simulink model "SkywalkerX8_Lateral_Control_Digital_Verification"  (R2018a)
settings: Solver=FixedStepAuto  StartTime=0.0  StopTime=30  FixedStep=0.001  RelTol=1e-3
undefined symbols (not defined in the file): DiscIntNeverNeededParam, sigbuilder_block, SkywalkerX8
libraries: simulink_extras x11, simulink x1
settings Model: SnapshotBufferSize=1000  SnapshotInterval=1  Creator=David  LastModifiedBy=David

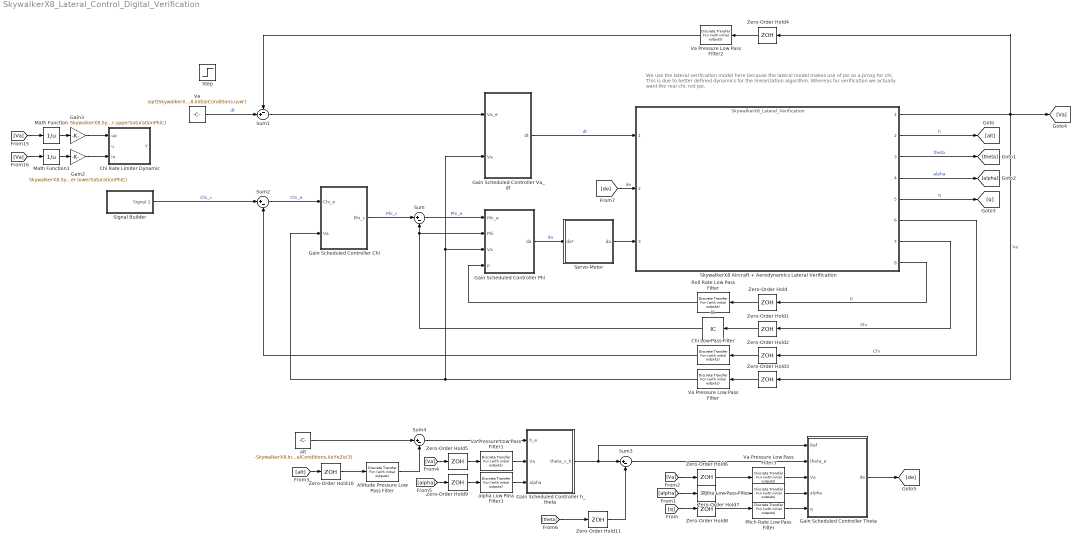
== system SkywalkerX8_Lateral_Control_Digital_Verification ==
  note: We use the lateral verification model here because the lateral model makes use of psi as a proxy for chi.
      | This is due to better defined dynamics for the linearization algorithm. Whereas for verification we actually
      | want the real chi, not psi.
  Altitude Pressure Low Pass Filter : simulink_extras/Additional Discrete/Discrete Transfer Fcn (with initial outputs)  N=cell2mat(SkywalkerX8.Sensors.Filters.AltitudePressure.FilterTFDigital.Numerator)  D=cell2mat(SkywalkerX8.Sensors.Filters.AltitudePressure.FilterTFDigital.Denominator)  U0=-SkywalkerX8.InitialConditions.XeYeZe(3)  Y0=-SkywalkerX8.InitialConditions.XeYeZe(3)  TS=SkywalkerX8.Sensors.Filters.AltitudePressure.FilterSampleTime
      settings: SourceProductName=Simulink  SourceProductBaseCode=SL
  Chi Low Pass Filter : simulink_extras/Additional Discrete/Discrete Transfer Fcn (with initial outputs)  N=cell2mat(SkywalkerX8.Sensors.EKF.GPSSmoothing.Filters.ChiFilter.TFDigital.Numerator)  D=cell2mat(SkywalkerX8.Sensors.EKF.GPSSmoothing.Filters.ChiFilter.TFDigital.Denominator)  U0=SkywalkerX8.Sensors.EKF.GPSSmoothing.Filters.ChiFilter.InitialCondition  Y0=SkywalkerX8.Sensors.EKF.GPSSmoothing.Filters.ChiFilter.InitialCondition  TS=SkywalkerX8.Sensors.EKF.GPSSmoothing.Filters.ChiFilter.SampleTime
      settings: SourceProductName=Simulink  SourceProductBaseCode=SL
  Chi Rate Limiter Dynamic : Subsystem  mask{initOutput=SkywalkerX8.InitialConditions.PhiThetaPsi(3)}
      mask prompts: initOutput "Initial output of dynamic rate limiter"
      mask DialogControl DescGroupVar Prompt: Rate Limiter Dynamic
      mask DialogControl DescTextVar Prompt: Limit rising and falling rates of the signals at the second input by using the first input (upper limit) and the third input (lower limit).
      mask Display:
      | image('rateLimit.png')
      | 
      | port_label('input', 1, 'up')
      | port_label('input', 2, 'u')
      | port_label('input', 3, 'lo')
      | 
      | port_label('output', 1, 'Y')
  Gain Scheduled Controller Chi : Subsystem
  Gain Scheduled Controller Phi : Subsystem
  Gain Scheduled Controller Theta : Subsystem
  Gain Scheduled Controller Va_dt : Subsystem
  Gain Scheduled Controller h_theta : Subsystem
  Gain2 : Gain  Gain=SkywalkerX8.System.Gravity*tan(0.75*SkywalkerX8.Control.Lateral.ChiController.lowerSaturationPhiC)
  Gain3 : Gain  Gain=SkywalkerX8.System.Gravity*tan(0.75*SkywalkerX8.Control.Lateral.ChiController.upperSaturationPhiC)
  IC : InitialCondition  Value=SkywalkerX8.InitialConditions.PhiThetaPsi(1)
  Math Function : Math  Operator=reciprocal  SaturateOnIntegerOverflow=on
  Math Function1 : Math  Operator=reciprocal  SaturateOnIntegerOverflow=on
  Pitch Rate Low Pass Filter : simulink_extras/Additional Discrete/Discrete Transfer Fcn (with initial outputs)  N=cell2mat(SkywalkerX8.Sensors.Filters.AngularRates.Pitch.FilterTFDigital.Numerator)  D=cell2mat(SkywalkerX8.Sensors.Filters.AngularRates.Pitch.FilterTFDigital.Denominator)  U0=SkywalkerX8.Sensors.Filters.AngularRates.Pitch.InitialCondition  Y0=SkywalkerX8.Sensors.Filters.AngularRates.Pitch.InitialCondition  TS=SkywalkerX8.Sensors.Filters.AngularRates.Pitch.FilterSampleTime
      settings: SourceProductName=Simulink  SourceProductBaseCode=SL
  Roll Rate Low Pass Filter : simulink_extras/Additional Discrete/Discrete Transfer Fcn (with initial outputs)  N=cell2mat(SkywalkerX8.Sensors.Filters.AngularRates.Roll.FilterTFDigital.Numerator)  D=cell2mat(SkywalkerX8.Sensors.Filters.AngularRates.Roll.FilterTFDigital.Denominator)  U0=SkywalkerX8.Sensors.Filters.AngularRates.Roll.InitialCondition  Y0=SkywalkerX8.Sensors.Filters.AngularRates.Roll.InitialCondition  TS=SkywalkerX8.Sensors.Filters.AngularRates.Roll.FilterSampleTime
      settings: SourceProductName=Simulink  SourceProductBaseCode=SL
  Servo-Motor : Subsystem
      mask Display: image('servo.jpg', 'center')
  Signal Builder : Subsystem  Tag=STV Subsys  LoadFcn=sigbuilder_block('load');  StartFcn=sigbuilder_block('start');  StopFcn=sigbuilder_block('stop');  ClipboardFcn=sigbuilder_block('clipboard');  mask(Sigbuilder block){tuvar=[0:10]}
      mask help: Simulink:masks:SigbuilderBlock_MD
      mask init:
      | if ~strcmp(get_param(bdroot(gcbh),'SimulationStatus'),'stopped') tuvar = sigbuilder_block('maskInit'); end
      settings: CopyFcn=sigbuilder_block('copy');  DeleteFcn=sigbuilder_block('delete');  ModelCloseFcn=sigbuilder_block('modelClose');  PreSaveFcn=sigbuilder_block('preSave');  PauseFcn=sigbuilder_block('pause');  ContinueFcn=sigbuilder_block('continue');  NameChangeFcn=sigbuilder_block('namechange');  OpenFcn=sigbuilder_block('open',[437.6 199.2 550.4 400 ]);  CloseFcn=sigbuilder_block('close');
      mask Display: plot(0, 0, 100, 100,[2, 2, 32, 32, 2], [68, 8, 8, 68, 68],[32, 2], [38, 38], [32, 19, 2],[53, 60, 44], [32, 17, 17, 2],[16, 16, 31, 31]);txt = getActiveGroup(gcbh);text(2, 100, txt,'verticalAlignment', 'top');
  SkywalkerX8 Aircraft + Aerodynamics Lateral Verification : ModelReference  ModelNameDialog=SkywalkerX8_Lateral_Verification.slx  ModelReferenceVersion=1.41
      mask Display:
      | image('x8SkySunset.png', 'center')
      | 
      | port_label('input', 1, '\delta_t (Unitless)', 'texmode', 'on')
      | port_label('input', 2, '\delta_e (rad)', 'texmode', 'on')
      | port_label('input', 3, '\delta_a (rad)', 'texmode', 'on')
      | 
      | port_label('output', 1, 'V_a (m/s)', 'texmode', 'on')
      | port_label('output', 2, 'Altitude (m)', 'texmode', 'on')
      | port_label('output', 3, '\theta (rad)', 'texmode', 'on')
      | port_label('output', 4, 'alpha (rad)', 'texmode', 'on')
      | port_label('output', 5, 'q (rad/s)', 'texmode', 'on')
      | port_label('output', 6, '\chi (rad)', 'texmode', 'on')
      | port_label('output', 7, '\Phi (rad)', 'texmode', 'on')
      | port_label('output', 8, 'p (rad/s)', 'texmode', 'on')
  Step : Step  After=deg2rad(90)  SampleTime=0
  Sum{,2..4} (4 alike) : Sum  Inputs=|+-
  Sum1 : Sum  Inputs=-+|
  Va : Constant  Value=sqrt(SkywalkerX8.InitialConditions.uvw*SkywalkerX8.InitialConditions.uvw')
  Va Pressure Low Pass Filter{,1..3} (4 alike) : simulink_extras/Additional Discrete/Discrete Transfer Fcn (with initial outputs)  N=cell2mat(SkywalkerX8.Sensors.Filters.AirspeedPressure.FilterTFDigital.Numerator)  D=cell2mat(SkywalkerX8.Sensors.Filters.AirspeedPressure.FilterTFDigital.Denominator)  U0=sqrt(SkywalkerX8.InitialConditions.uvw*SkywalkerX8.InitialConditions.uvw')  Y0=SkywalkerX8.Sensors.Filters.AirspeedPressure.InitialCondition  TS=SkywalkerX8.Sensors.Filters.AirspeedPressure.FilterSampleTime
      settings: SourceProductName=Simulink  SourceProductBaseCode=SL
  Zero-Order Hold : ZeroOrderHold  SampleTime=SkywalkerX8.Sensors.IMU.Gyroscope.SampleTime
  Zero-Order Hold1 : ZeroOrderHold  SampleTime=SkywalkerX8.Sensors.EKF.Attitude.StateTransitionSampleTime
  Zero-Order Hold10 : ZeroOrderHold  SampleTime=SkywalkerX8.Sensors.AltitudePressure.SampleTime
  Zero-Order Hold11 : ZeroOrderHold  SampleTime=SkywalkerX8.Sensors.EKF.GPSSmoothing.StateTransitionSampleTime
  Zero-Order Hold2 : ZeroOrderHold  SampleTime=SkywalkerX8.Sensors.EKF.GPSSmoothing.MeasurementSampleTime
  Zero-Order Hold{3..6} (4 alike) : ZeroOrderHold  SampleTime=SkywalkerX8.Sensors.AirspeedPressure.SampleTime
  Zero-Order Hold7 : ZeroOrderHold  SampleTime=SkywalkerX8.Sensors.AoA.SampleTime
  Zero-Order Hold8 : ZeroOrderHold  SampleTime=SkywalkerX8.Sensors.IMU.Gyroscope.SampleTime
  Zero-Order Hold9 : ZeroOrderHold  SampleTime=SkywalkerX8.Sensors.AoA.SampleTime
  alpha Low Pass Filter : simulink_extras/Additional Discrete/Discrete Transfer Fcn (with initial outputs)  N=cell2mat(SkywalkerX8.Sensors.Filters.AoA.FilterTFDigital.Numerator)  D=cell2mat(SkywalkerX8.Sensors.Filters.AoA.FilterTFDigital.Denominator)  U0=SkywalkerX8.Sensors.Filters.AoA.InitialCondition  Y0=SkywalkerX8.Sensors.Filters.AoA.InitialCondition  TS=SkywalkerX8.Sensors.Filters.AoA.FilterSampleTime
      settings: SourceProductName=Simulink  SourceProductBaseCode=SL
  alpha Low Pass Filter1 : simulink_extras/Additional Discrete/Discrete Transfer Fcn (with initial outputs)  N=cell2mat(SkywalkerX8.Sensors.Filters.AoA.FilterTFDigital.Numerator)  D=cell2mat(SkywalkerX8.Sensors.Filters.AoA.FilterTFDigital.Denominator)  U0=SkywalkerX8.Sensors.Filters.AoA.InitialCondition  Y0=SkywalkerX8.Sensors.Filters.AoA.InitialCondition  TS=SkywalkerX8.Sensors.Filters.AoA.FilterSampleTime
      settings: SourceProductName=Simulink  SourceProductBaseCode=SL
  alt : Constant  Value=-SkywalkerX8.InitialConditions.XeYeZe(3)
  wires:
  SkywalkerX8 Aircraft + Aerodynamics Lateral Verification/7 -> Zero-Order Hold1/1  "Phi"
  SkywalkerX8 Aircraft + Aerodynamics Lateral Verification/1 -> [Va], Zero-Order Hold3/1, Zero-Order Hold4/1  "Va"
  Gain Scheduled Controller Chi/1(Phi_c) -> Sum/1  "Phi_c"
  Sum/1 -> Gain Scheduled Controller Phi/1(Phi_e)  "Phi_e"
  Sum2/1 -> Gain Scheduled Controller Chi/1(Chi_e)  "Chi_e"
  SkywalkerX8 Aircraft + Aerodynamics Lateral Verification/8 -> Zero-Order Hold/1  "p"
  Gain Scheduled Controller Phi/1(da) -> Servo-Motor/1(da*)  "da"
  [de] -> SkywalkerX8 Aircraft + Aerodynamics Lateral Verification/2  "de"
  Gain Scheduled Controller Va_dt/1(dt) -> SkywalkerX8 Aircraft + Aerodynamics Lateral Verification/1  "dt"
  SkywalkerX8 Aircraft + Aerodynamics Lateral Verification/6 -> Zero-Order Hold2/1  "Chi"
  Va/1 -> Sum1/2  "dt"
  Sum1/1 -> Gain Scheduled Controller Va_dt/1(Va_e)
  Gain Scheduled Controller h_theta/1(theta_c_h) -> Gain Scheduled Controller Theta/1(Ref), Sum3/1
  Sum3/1 -> Gain Scheduled Controller Theta/2(theta_e)
  SkywalkerX8 Aircraft + Aerodynamics Lateral Verification/2 -> [alt]  "h"
  SkywalkerX8 Aircraft + Aerodynamics Lateral Verification/3 -> [theta]  "theta"
  SkywalkerX8 Aircraft + Aerodynamics Lateral Verification/4 -> [alpha]  "alpha"
  SkywalkerX8 Aircraft + Aerodynamics Lateral Verification/5 -> [q]  "q"
  [q] -> Zero-Order Hold8/1
  [alpha] -> Zero-Order Hold7/1
  [Va] -> Zero-Order Hold6/1
  Sum4/1 -> Gain Scheduled Controller h_theta/1(h_e)
  [alt] -> Zero-Order Hold10/1
  alt/1 -> Sum4/1
  [Va] -> Zero-Order Hold5/1
  [alpha] -> Zero-Order Hold9/1
  [theta] -> Zero-Order Hold11/1
  Gain Scheduled Controller Theta/1(de) -> [de]
  Servo-Motor/1(da) -> SkywalkerX8 Aircraft + Aerodynamics Lateral Verification/3
  Zero-Order Hold/1 -> Roll Rate Low Pass Filter/1
  Zero-Order Hold1/1 -> IC/1
  Zero-Order Hold2/1 -> Chi Low Pass Filter/1
  Zero-Order Hold3/1 -> Va Pressure Low Pass Filter/1
  Zero-Order Hold4/1 -> Va Pressure Low Pass Filter2/1
  Zero-Order Hold5/1 -> Va Pressure Low Pass Filter1/1
  Zero-Order Hold6/1 -> Va Pressure Low Pass Filter3/1
  Zero-Order Hold7/1 -> alpha Low Pass Filter/1
  Zero-Order Hold8/1 -> Pitch Rate Low Pass Filter/1
  Zero-Order Hold9/1 -> alpha Low Pass Filter1/1
  Zero-Order Hold10/1 -> Altitude Pressure Low Pass Filter/1
  Zero-Order Hold11/1 -> Sum3/2
  Roll Rate Low Pass Filter/1 -> Gain Scheduled Controller Phi/4(p)
  Chi Low Pass Filter/1 -> Sum2/2
  Va Pressure Low Pass Filter/1 -> Gain Scheduled Controller Chi/2(Va), Gain Scheduled Controller Va_dt/2(Va), Gain Scheduled Controller Phi/3(Va)
  Pitch Rate Low Pass Filter/1 -> Gain Scheduled Controller Theta/5(q)
  alpha Low Pass Filter/1 -> Gain Scheduled Controller Theta/4(alpha)
  Altitude Pressure Low Pass Filter/1 -> Sum4/2
  Va Pressure Low Pass Filter1/1 -> Gain Scheduled Controller h_theta/2(Va)
  alpha Low Pass Filter1/1 -> Gain Scheduled Controller h_theta/3(alpha)
  Va Pressure Low Pass Filter2/1 -> Sum1/1
  Va Pressure Low Pass Filter3/1 -> Gain Scheduled Controller Theta/3(Va)
  IC/1 -> Gain Scheduled Controller Phi/2(Phi), Sum/2
  [Va] -> Math Function/1
  Math Function1/1 -> Gain2/1
  Gain2/1 -> Chi Rate Limiter Dynamic/3(lo)
  Math Function/1 -> Gain3/1
  Gain3/1 -> Chi Rate Limiter Dynamic/1(up)
  [Va] -> Math Function1/1
  Signal Builder/1(Signal 1) -> Sum2/1  "Chi_c"

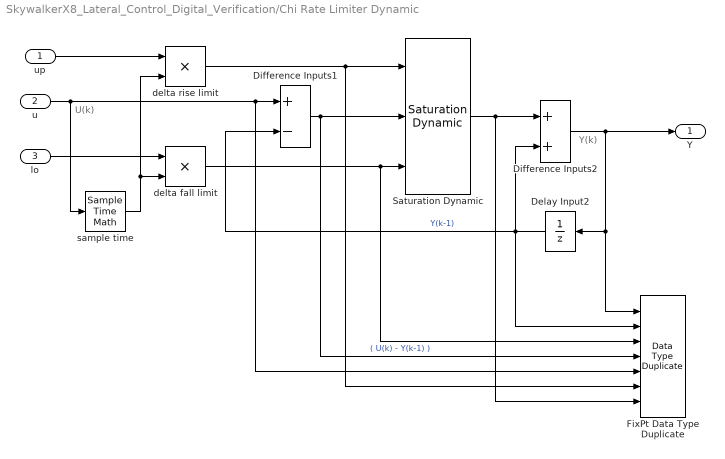
== system SkywalkerX8_Lateral_Control_Digital_Verification/Chi Rate Limiter Dynamic ==
  note: U(k)
  note: Y(k)
  up : Inport
  u : Inport  Port=2
  lo : Inport  Port=3
  Delay Input2 : UnitDelay  Description=Store in Global RAM  DisableCoverage=on  InitialCondition=initOutput  SampleTime=-1
  Difference Inputs1 : Sum  Description=Add in CPU  DisableCoverage=on  Inputs=+-  OutDataTypeStr=Inherit: Inherit via back propagation
  Difference Inputs2 : Sum  Description=Add in CPU  OutDataTypeStr=Inherit: Inherit via back propagation
  FixPt Data Type Duplicate : DataTypeDuplicate  DisableCoverage=on  NumInputPorts=7
  Saturation Dynamic : simulink/Discontinuities/Saturation Dynamic  OutMin=[]  OutMax=[]  OutDataTypeStr=Inherit: Same as second input  OutDataType=fixdt(1, 16)  OutScaling=2^-10  DoSatur=off
  delta fall limit : Product  DisableCoverage=on  Inputs=**  OutDataTypeStr=Inherit: Inherit via back propagation  SaturateOnIntegerOverflow=on
  delta rise limit : Product  DisableCoverage=on  Inputs=**  OutDataTypeStr=Inherit: Inherit via back propagation  SaturateOnIntegerOverflow=on
  sample time : SampleTimeMath  DisableCoverage=on  TsampMathOp=Ts Only  weightValue=1
  Y : Outport  InitialOutput=0
  wires:
  Delay Input2/1 -> Difference Inputs1/2, FixPt Data Type Duplicate/2, Difference Inputs2/2  "Y(k-1)"
  Difference Inputs1/1 -> FixPt Data Type Duplicate/4, Saturation Dynamic/2  "( U(k) - Y(k-1) )"
  Difference Inputs2/1 -> Y/1, Delay Input2/1, FixPt Data Type Duplicate/1
  u/1 -> Difference Inputs1/1, FixPt Data Type Duplicate/5, sample time/1
  delta fall limit/1 -> FixPt Data Type Duplicate/3, Saturation Dynamic/3
  sample time/1 -> delta fall limit/2, delta rise limit/2
  Saturation Dynamic/1 -> Difference Inputs2/1, FixPt Data Type Duplicate/7
  delta rise limit/1 -> FixPt Data Type Duplicate/6, Saturation Dynamic/1
  lo/1 -> delta fall limit/1
  up/1 -> delta rise limit/1

== system SkywalkerX8_Lateral_Control_Digital_Verification/Gain Scheduled Controller Chi ==
  Chi_e : Inport
  Va : Inport  Port=2
  PIDF Controller Chi Ki 2D Lookup Table : Lookup_n-D  NumberOfTableDimensions=1  BreakpointsForDimension1=SkywalkerX8.Control.Lateral.SchedulingVariables.VaArray  BreakpointsForDimension2=SkywalkerX8.Control.Longitudinal.SchedulingVariables.alphaArray  Table=SkywalkerX8.Control.Lateral.ChiController.Digital.KiChi  InternalRulePriority=Speed  RndMeth=Simplest  InputSameDT=on
  PIDF Controller Chi Kp 2D Lookup Table : Lookup_n-D  NumberOfTableDimensions=1  BreakpointsForDimension1=SkywalkerX8.Control.Lateral.SchedulingVariables.VaArray  BreakpointsForDimension2=SkywalkerX8.Control.Longitudinal.SchedulingVariables.alphaArray  Table=SkywalkerX8.Control.Lateral.ChiController.Digital.KpChi  InternalRulePriority=Speed  RndMeth=Simplest  InputSameDT=on
  PIDF Controller Va_theta : Subsystem
  Saturation : Saturate  UpperLimit=SkywalkerX8.Control.Lateral.ChiController.upperSaturationPhiC  LowerLimit=SkywalkerX8.Control.Lateral.ChiController.lowerSaturationPhiC
  Phi_c : Outport
  wires:
  PIDF Controller Chi Kp 2D Lookup Table/1 -> PIDF Controller Va_theta/2(P)
  Chi_e/1 -> PIDF Controller Va_theta/1(u)
  Va/1 -> PIDF Controller Chi Kp 2D Lookup Table/1, PIDF Controller Chi Ki 2D Lookup Table/1
  PIDF Controller Chi Ki 2D Lookup Table/1 -> PIDF Controller Va_theta/3(I)
  Saturation/1 -> PIDF Controller Va_theta/4(Post-Saturation), Phi_c/1
  PIDF Controller Va_theta/1(y) -> PIDF Controller Va_theta/5(Pre-Saturation), Saturation/1

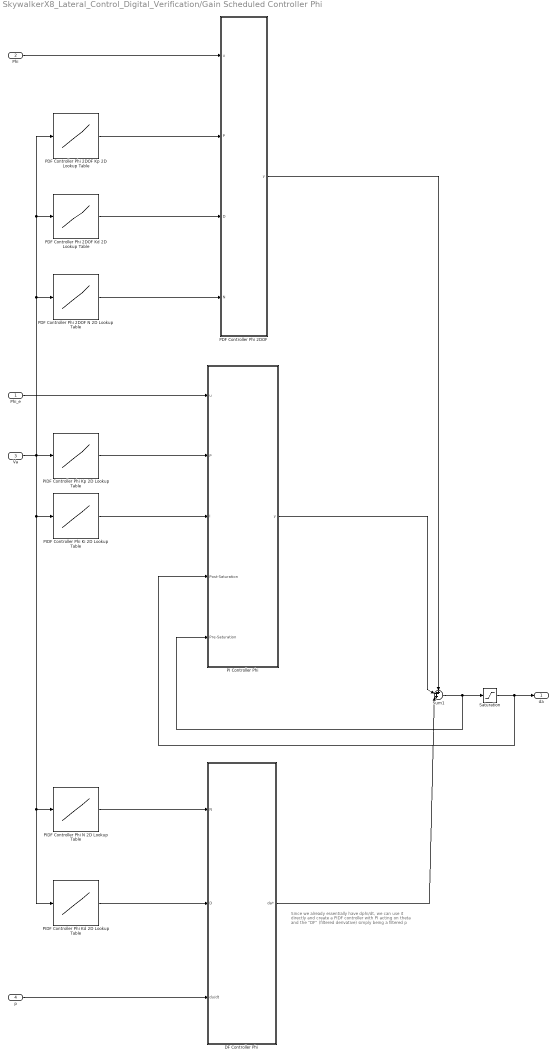
== system SkywalkerX8_Lateral_Control_Digital_Verification/Gain Scheduled Controller Phi ==
  note: Since we already essentially have dphi/dt,
      | we can use it directly and create a PIDF controller
      | with PI acting on theta and the "DF" (filtered derivative)
      | simply being a filtered p
  Phi_e : Inport
  Phi : Inport  Port=2
  Va : Inport  Port=3
  p : Inport  Port=4
  DF Controller Phi : Subsystem
  PDF Controller Phi 2DOF : Subsystem
  PDF Controller Phi 2DOF Kd 2D Lookup Table : Lookup_n-D  NumberOfTableDimensions=1  BreakpointsForDimension1=SkywalkerX8.Control.Lateral.SchedulingVariables.VaArray  BreakpointsForDimension2=SkywalkerX8.Control.Longitudinal.SchedulingVariables.alphaArray  Table=SkywalkerX8.Control.Lateral.PhiController.Digital.KdPhi2DOF  InternalRulePriority=Speed  RndMeth=Simplest  InputSameDT=on
  PDF Controller Phi 2DOF Kp 2D Lookup Table : Lookup_n-D  NumberOfTableDimensions=1  BreakpointsForDimension1=SkywalkerX8.Control.Lateral.SchedulingVariables.VaArray  BreakpointsForDimension2=SkywalkerX8.Control.Longitudinal.SchedulingVariables.alphaArray  Table=SkywalkerX8.Control.Lateral.PhiController.Digital.KpPhi2DOF  InternalRulePriority=Speed  RndMeth=Simplest  InputSameDT=on
  PDF Controller Phi 2DOF N 2D Lookup Table : Lookup_n-D  NumberOfTableDimensions=1  BreakpointsForDimension1=SkywalkerX8.Control.Lateral.SchedulingVariables.VaArray  BreakpointsForDimension2=SkywalkerX8.Control.Longitudinal.SchedulingVariables.alphaArray  Table=SkywalkerX8.Control.Lateral.PhiController.Digital.NPhi2DOF  InternalRulePriority=Speed  RndMeth=Simplest  InputSameDT=on
  PI Controller Phi : Subsystem
  PIDF Controller Phi Kd 2D Lookup Table : Lookup_n-D  NumberOfTableDimensions=1  BreakpointsForDimension1=SkywalkerX8.Control.Lateral.SchedulingVariables.VaArray  BreakpointsForDimension2=SkywalkerX8.Control.Longitudinal.SchedulingVariables.alphaArray  Table=SkywalkerX8.Control.Lateral.PhiController.Digital.KdPhi  InternalRulePriority=Speed  RndMeth=Simplest  InputSameDT=on
  PIDF Controller Phi Ki 2D Lookup Table : Lookup_n-D  NumberOfTableDimensions=1  BreakpointsForDimension1=SkywalkerX8.Control.Lateral.SchedulingVariables.VaArray  BreakpointsForDimension2=SkywalkerX8.Control.Longitudinal.SchedulingVariables.alphaArray  Table=SkywalkerX8.Control.Lateral.PhiController.Digital.KiPhi  InternalRulePriority=Speed  RndMeth=Simplest  InputSameDT=on
  PIDF Controller Phi Kp 2D Lookup Table : Lookup_n-D  NumberOfTableDimensions=1  BreakpointsForDimension1=SkywalkerX8.Control.Lateral.SchedulingVariables.VaArray  BreakpointsForDimension2=SkywalkerX8.Control.Longitudinal.SchedulingVariables.alphaArray  Table=SkywalkerX8.Control.Lateral.PhiController.Digital.KpPhi  InternalRulePriority=Speed  RndMeth=Simplest  InputSameDT=on
  PIDF Controller Phi N 2D Lookup Table : Lookup_n-D  NumberOfTableDimensions=1  BreakpointsForDimension1=SkywalkerX8.Control.Lateral.SchedulingVariables.VaArray  BreakpointsForDimension2=SkywalkerX8.Control.Longitudinal.SchedulingVariables.alphaArray  Table=SkywalkerX8.Control.Lateral.PhiController.Digital.NPhi  InternalRulePriority=Speed  RndMeth=Simplest  InputSameDT=on
  Saturation : Saturate  UpperLimit=SkywalkerX8.Control.Lateral.PhiController.upperSaturationDa  LowerLimit=SkywalkerX8.Control.Lateral.PhiController.lowerSaturationDa
  Sum1 : Sum  Inputs=+++|
  da : Outport
  wires:
  Va/1 -> PDF Controller Phi 2DOF Kp 2D Lookup Table/1, PDF Controller Phi 2DOF Kd 2D Lookup Table/1, PDF Controller Phi 2DOF N 2D Lookup Table/1, PIDF Controller Phi N 2D Lookup Table/1, PIDF Controller Phi Kd 2D Lookup Table/1, PIDF Controller Phi Ki 2D Lookup Table/1, PIDF Controller Phi Kp 2D Lookup Table/1
  Phi_e/1 -> PI Controller Phi/1(u)
  PIDF Controller Phi Kp 2D Lookup Table/1 -> PI Controller Phi/2(P)
  PIDF Controller Phi Ki 2D Lookup Table/1 -> PI Controller Phi/3(I)
  PI Controller Phi/1(y) -> Sum1/2
  Sum1/1 -> Saturation/1, PI Controller Phi/5(Pre-Saturation)
  p/1 -> DF Controller Phi/3(du/dt)
  DF Controller Phi/1(da*) -> Sum1/3
  PIDF Controller Phi N 2D Lookup Table/1 -> DF Controller Phi/1(N)
  PIDF Controller Phi Kd 2D Lookup Table/1 -> DF Controller Phi/2(D)
  Saturation/1 -> da/1, PI Controller Phi/4(Post-Saturation)
  PDF Controller Phi 2DOF Kp 2D Lookup Table/1 -> PDF Controller Phi 2DOF/2(P)
  PDF Controller Phi 2DOF Kd 2D Lookup Table/1 -> PDF Controller Phi 2DOF/3(D)
  PDF Controller Phi 2DOF N 2D Lookup Table/1 -> PDF Controller Phi 2DOF/4(N)
  Phi/1 -> PDF Controller Phi 2DOF/1(u)
  PDF Controller Phi 2DOF/1(y) -> Sum1/1

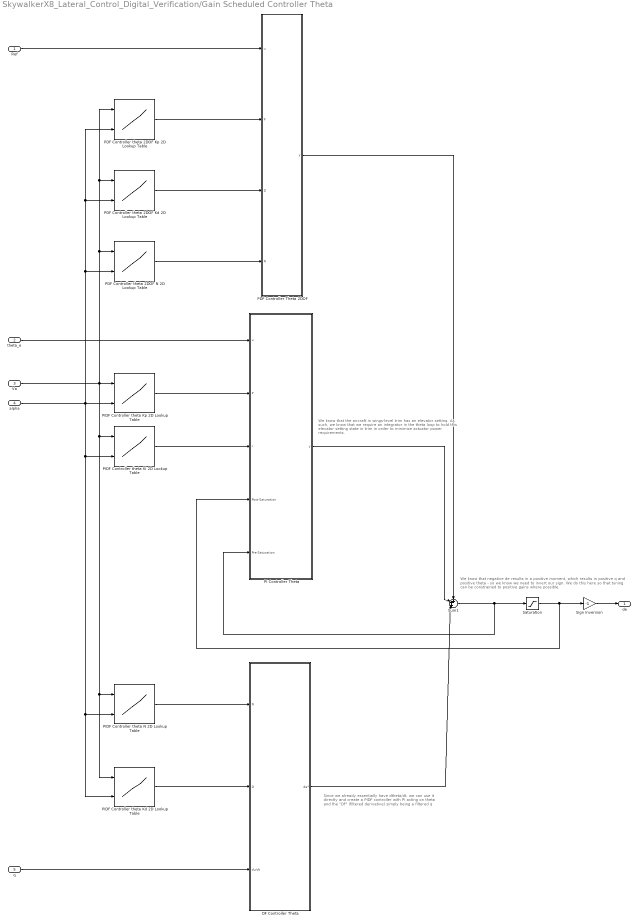
== system SkywalkerX8_Lateral_Control_Digital_Verification/Gain Scheduled Controller Theta ==
  note: Since we already essentially have dtheta/dt,
      | we can use it directly and create a PIDF controller
      | with PI acting on theta and the "DF" (filtered derivative)
      | simply being a filtered q
  note: We know that negative de results in a positive moment, which results in
      | positive q and positive theta - so we know we need to invert our sign.
      | We do this here so that tuning can be constrained to positive gains where possible.
  note: We know that the aircraft in wings-level trim has an elevator setting. As such, we know that we require an integrator in the theta loop to hold this elevator setting state in trim in order to minimize actuator power requirements.
  Ref : Inport
  theta_e : Inport  Port=2
  Va : Inport  Port=3
  alpha : Inport  Port=4
  q : Inport  Port=5
  DF Controller Theta : Subsystem
  PDF Controller Theta 2DOF : Subsystem
  PDF Controller theta 2DOF Kd 2D Lookup Table : Lookup_n-D  BreakpointsForDimension1=SkywalkerX8.Control.Longitudinal.SchedulingVariables.VaArray  BreakpointsForDimension2=SkywalkerX8.Control.Longitudinal.SchedulingVariables.alphaArray  Table=SkywalkerX8.Control.Longitudinal.thetaController.Digital.KdTheta2DOF  InternalRulePriority=Speed  RndMeth=Simplest  InputSameDT=on
  PDF Controller theta 2DOF Kp 2D Lookup Table : Lookup_n-D  BreakpointsForDimension1=SkywalkerX8.Control.Longitudinal.SchedulingVariables.VaArray  BreakpointsForDimension2=SkywalkerX8.Control.Longitudinal.SchedulingVariables.alphaArray  Table=SkywalkerX8.Control.Longitudinal.thetaController.Digital.KpTheta2DOF  InternalRulePriority=Speed  RndMeth=Simplest  InputSameDT=on
  PDF Controller theta 2DOF N 2D Lookup Table : Lookup_n-D  BreakpointsForDimension1=SkywalkerX8.Control.Longitudinal.SchedulingVariables.VaArray  BreakpointsForDimension2=SkywalkerX8.Control.Longitudinal.SchedulingVariables.alphaArray  Table=SkywalkerX8.Control.Longitudinal.thetaController.Digital.NTheta2DOF  InternalRulePriority=Speed  RndMeth=Simplest  InputSameDT=on
  PI Controller Theta : Subsystem
  PIDF Controller theta Kd 2D Lookup Table : Lookup_n-D  BreakpointsForDimension1=SkywalkerX8.Control.Longitudinal.SchedulingVariables.VaArray  BreakpointsForDimension2=SkywalkerX8.Control.Longitudinal.SchedulingVariables.alphaArray  Table=SkywalkerX8.Control.Longitudinal.thetaController.Digital.KdTheta  InternalRulePriority=Speed  RndMeth=Simplest  InputSameDT=on
  PIDF Controller theta Ki 2D Lookup Table : Lookup_n-D  BreakpointsForDimension1=SkywalkerX8.Control.Longitudinal.SchedulingVariables.VaArray  BreakpointsForDimension2=SkywalkerX8.Control.Longitudinal.SchedulingVariables.alphaArray  Table=SkywalkerX8.Control.Longitudinal.thetaController.Digital.KiTheta  InternalRulePriority=Speed  RndMeth=Simplest  InputSameDT=on
  PIDF Controller theta Kp 2D Lookup Table : Lookup_n-D  BreakpointsForDimension1=SkywalkerX8.Control.Longitudinal.SchedulingVariables.VaArray  BreakpointsForDimension2=SkywalkerX8.Control.Longitudinal.SchedulingVariables.alphaArray  Table=SkywalkerX8.Control.Longitudinal.thetaController.Digital.KpTheta  InternalRulePriority=Speed  RndMeth=Simplest  InputSameDT=on
  PIDF Controller theta N 2D Lookup Table : Lookup_n-D  BreakpointsForDimension1=SkywalkerX8.Control.Longitudinal.SchedulingVariables.VaArray  BreakpointsForDimension2=SkywalkerX8.Control.Longitudinal.SchedulingVariables.alphaArray  Table=SkywalkerX8.Control.Longitudinal.thetaController.Digital.NTheta  InternalRulePriority=Speed  RndMeth=Simplest  InputSameDT=on
  Saturation : Saturate  UpperLimit=SkywalkerX8.Control.Longitudinal.thetaController.Digital.upperSaturationNegativeDe  LowerLimit=SkywalkerX8.Control.Longitudinal.thetaController.Digital.lowerSaturationNegativeDe
  Sign Inversion : Gain  Gain=-1
  Sum1 : Sum  Inputs=+++|
  de : Outport
  wires:
  Va/1 -> PDF Controller theta 2DOF Kd 2D Lookup Table/1, PDF Controller theta 2DOF Kp 2D Lookup Table/1, PDF Controller theta 2DOF N 2D Lookup Table/1, PIDF Controller theta N 2D Lookup Table/1, PIDF Controller theta Kd 2D Lookup Table/1, PIDF Controller theta Ki 2D Lookup Table/1, PIDF Controller theta Kp 2D Lookup Table/1
  theta_e/1 -> PI Controller Theta/1(u)
  PIDF Controller theta Kp 2D Lookup Table/1 -> PI Controller Theta/2(P)
  PIDF Controller theta Ki 2D Lookup Table/1 -> PI Controller Theta/3(I)
  alpha/1 -> PDF Controller theta 2DOF N 2D Lookup Table/2, PDF Controller theta 2DOF Kd 2D Lookup Table/2, PDF Controller theta 2DOF Kp 2D Lookup Table/2, PIDF Controller theta N 2D Lookup Table/2, PIDF Controller theta Kd 2D Lookup Table/2, PIDF Controller theta Ki 2D Lookup Table/2, PIDF Controller theta Kp 2D Lookup Table/2
  PI Controller Theta/1(y) -> Sum1/2
  Sum1/1 -> Saturation/1, PI Controller Theta/5(Pre-Saturation)
  Saturation/1 -> Sign Inversion/1, PI Controller Theta/4(Post-Saturation)
  PIDF Controller theta N 2D Lookup Table/1 -> DF Controller Theta/1(N)
  PIDF Controller theta Kd 2D Lookup Table/1 -> DF Controller Theta/2(D)
  q/1 -> DF Controller Theta/3(du/dt)
  DF Controller Theta/1(de*) -> Sum1/3
  Sign Inversion/1 -> de/1
  PDF Controller theta 2DOF Kp 2D Lookup Table/1 -> PDF Controller Theta 2DOF/2(P)
  PDF Controller theta 2DOF Kd 2D Lookup Table/1 -> PDF Controller Theta 2DOF/3(D)
  PDF Controller theta 2DOF N 2D Lookup Table/1 -> PDF Controller Theta 2DOF/4(N)
  Ref/1 -> PDF Controller Theta 2DOF/1(u)
  PDF Controller Theta 2DOF/1(y) -> Sum1/1

== system SkywalkerX8_Lateral_Control_Digital_Verification/Gain Scheduled Controller Va_dt ==
  Va_e : Inport
  Va : Inport  Port=2
  PIDF Controller Va_dt : Subsystem
  PIDF Controller Va_dt Kd Lookup Table : Lookup_n-D  NumberOfTableDimensions=1  BreakpointsForDimension1=SkywalkerX8.Control.Longitudinal.SchedulingVariables.VaArray  BreakpointsForDimension2=[1 2 3 4 5]  Table=SkywalkerX8.Control.Longitudinal.VaDtController.Digital.KdVaDt  InternalRulePriority=Speed  RndMeth=Simplest  InputSameDT=on
  PIDF Controller Va_dt Ki Lookup Table : Lookup_n-D  NumberOfTableDimensions=1  BreakpointsForDimension1=SkywalkerX8.Control.Longitudinal.SchedulingVariables.VaArray  BreakpointsForDimension2=[1 2 3 4 5]  Table=SkywalkerX8.Control.Longitudinal.VaDtController.Digital.KiVaDt  InternalRulePriority=Speed  RndMeth=Simplest  InputSameDT=on
  PIDF Controller Va_dt Kp Lookup Table : Lookup_n-D  NumberOfTableDimensions=1  BreakpointsForDimension1=SkywalkerX8.Control.Longitudinal.SchedulingVariables.VaArray  BreakpointsForDimension2=[1 2 3 4 5]  Table=SkywalkerX8.Control.Longitudinal.VaDtController.Digital.KpVaDt  InternalRulePriority=Speed  RndMeth=Simplest  InputSameDT=on
  PIDF Controller Va_dt N Lookup Table : Lookup_n-D  NumberOfTableDimensions=1  BreakpointsForDimension1=SkywalkerX8.Control.Longitudinal.SchedulingVariables.VaArray  BreakpointsForDimension2=[1 2 3 4 5]  Table=SkywalkerX8.Control.Longitudinal.VaDtController.Digital.NVaDt  InternalRulePriority=Speed  RndMeth=Simplest  InputSameDT=on
  Saturation : Saturate  UpperLimit=SkywalkerX8.Control.Longitudinal.VaDtController.upperSaturationDt  LowerLimit=SkywalkerX8.Control.Longitudinal.VaDtController.lowerSaturationDt
  dt : Outport
  wires:
  Va_e/1 -> PIDF Controller Va_dt/1(u)
  Saturation/1 -> PIDF Controller Va_dt/6(Post-Saturation), dt/1
  PIDF Controller Va_dt Kp Lookup Table/1 -> PIDF Controller Va_dt/2(P)
  Va/1 -> PIDF Controller Va_dt Kp Lookup Table/1, PIDF Controller Va_dt N Lookup Table/1, PIDF Controller Va_dt Kd Lookup Table/1, PIDF Controller Va_dt Ki Lookup Table/1
  PIDF Controller Va_dt Ki Lookup Table/1 -> PIDF Controller Va_dt/3(I)
  PIDF Controller Va_dt Kd Lookup Table/1 -> PIDF Controller Va_dt/4(D)
  PIDF Controller Va_dt N Lookup Table/1 -> PIDF Controller Va_dt/5(N)
  PIDF Controller Va_dt/1(y) -> Saturation/1, PIDF Controller Va_dt/7(Pre-Saturation)

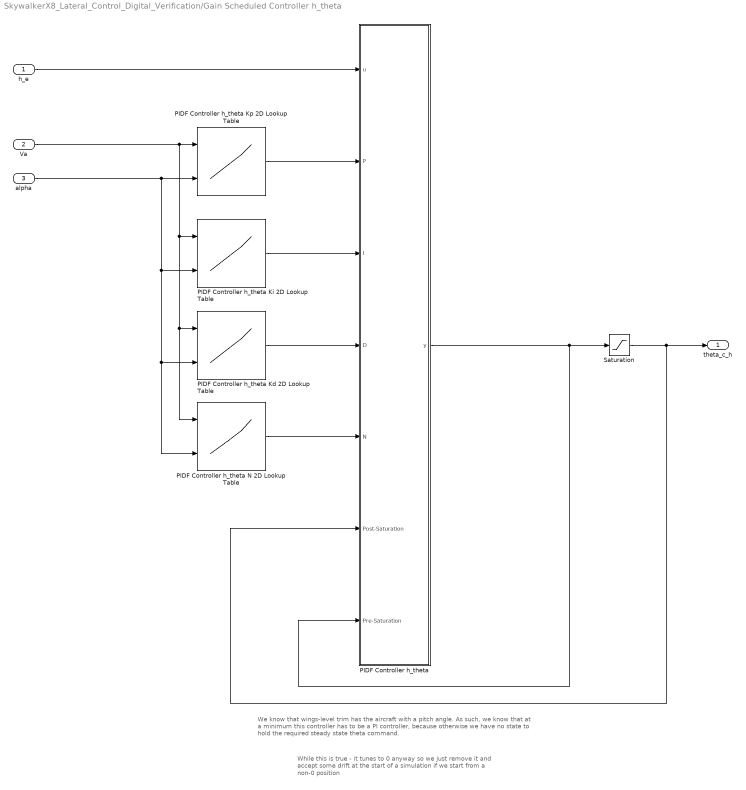
== system SkywalkerX8_Lateral_Control_Digital_Verification/Gain Scheduled Controller h_theta ==
  note: While this is true - it tunes to 0 anyway so we just remove it
      | and accept some drift at the start of a simulation if we start
      | from a non-0 position
  note: We know that wings-level trim has the aircraft with a pitch angle. As such,
      | we know that at a minimum this controller has to be a PI controller, because otherwise
      | we have no state to hold the required steady state theta command.
  h_e : Inport
  Va : Inport  Port=2
  alpha : Inport  Port=3
  PIDF Controller h_theta : Subsystem
  PIDF Controller h_theta Kd 2D Lookup Table : Lookup_n-D  BreakpointsForDimension1=SkywalkerX8.Control.Longitudinal.SchedulingVariables.VaArray  BreakpointsForDimension2=SkywalkerX8.Control.Longitudinal.SchedulingVariables.alphaArray  Table=SkywalkerX8.Control.Longitudinal.altController.Digital.KdAlt  InternalRulePriority=Speed  RndMeth=Simplest  InputSameDT=on
  PIDF Controller h_theta Ki 2D Lookup Table : Lookup_n-D  BreakpointsForDimension1=SkywalkerX8.Control.Longitudinal.SchedulingVariables.VaArray  BreakpointsForDimension2=SkywalkerX8.Control.Longitudinal.SchedulingVariables.alphaArray  Table=SkywalkerX8.Control.Longitudinal.altController.Digital.KiAlt  InternalRulePriority=Speed  RndMeth=Simplest  InputSameDT=on
  PIDF Controller h_theta Kp 2D Lookup Table : Lookup_n-D  BreakpointsForDimension1=SkywalkerX8.Control.Longitudinal.SchedulingVariables.VaArray  BreakpointsForDimension2=SkywalkerX8.Control.Longitudinal.SchedulingVariables.alphaArray  Table=SkywalkerX8.Control.Longitudinal.altController.Digital.KpAlt  InternalRulePriority=Speed  RndMeth=Simplest  InputSameDT=on
  PIDF Controller h_theta N 2D Lookup Table : Lookup_n-D  BreakpointsForDimension1=SkywalkerX8.Control.Longitudinal.SchedulingVariables.VaArray  BreakpointsForDimension2=SkywalkerX8.Control.Longitudinal.SchedulingVariables.alphaArray  Table=SkywalkerX8.Control.Longitudinal.altController.Digital.NAlt  InternalRulePriority=Speed  RndMeth=Simplest  InputSameDT=on
  Saturation : Saturate  UpperLimit=SkywalkerX8.Control.Longitudinal.altController.Digital.upperSaturationThetaC  LowerLimit=SkywalkerX8.Control.Longitudinal.altController.Digital.lowerSaturationThetaC
  theta_c_h : Outport
  wires:
  PIDF Controller h_theta Kp 2D Lookup Table/1 -> PIDF Controller h_theta/2(P)
  alpha/1 -> PIDF Controller h_theta N 2D Lookup Table/2, PIDF Controller h_theta Kd 2D Lookup Table/2, PIDF Controller h_theta Ki 2D Lookup Table/2, PIDF Controller h_theta Kp 2D Lookup Table/2
  h_e/1 -> PIDF Controller h_theta/1(u)
  Va/1 -> PIDF Controller h_theta N 2D Lookup Table/1, PIDF Controller h_theta Kd 2D Lookup Table/1, PIDF Controller h_theta Ki 2D Lookup Table/1, PIDF Controller h_theta Kp 2D Lookup Table/1
  PIDF Controller h_theta Kd 2D Lookup Table/1 -> PIDF Controller h_theta/4(D)
  PIDF Controller h_theta N 2D Lookup Table/1 -> PIDF Controller h_theta/5(N)
  Saturation/1 -> PIDF Controller h_theta/6(Post-Saturation), theta_c_h/1
  PIDF Controller h_theta/1(y) -> PIDF Controller h_theta/7(Pre-Saturation), Saturation/1
  PIDF Controller h_theta Ki 2D Lookup Table/1 -> PIDF Controller h_theta/3(I)

== system SkywalkerX8_Lateral_Control_Digital_Verification/Servo-Motor ==
  da* : Inport
  Rate Limiter : RateLimiter  Commented=through  RisingSlewLimit=SkywalkerX8.Actuators.Servos.RateLimit  FallingSlewLimit=-SkywalkerX8.Actuators.Servos.RateLimit  SampleTimeMode=inherited  InitialCondition=SkywalkerX8.InitialConditions.de
  Saturation : Saturate  UpperLimit=2*SkywalkerX8.Actuators.Servos.UpperSaturation  LowerLimit=2*SkywalkerX8.Actuators.Servos.LowerSaturation
  Transfer Fcn (with initial outputs) : simulink_extras/Additional Linear/Transfer Fcn (with initial outputs)  N=cell2mat(SkywalkerX8.Actuators.Servos.TF.Numerator)  D=cell2mat(SkywalkerX8.Actuators.Servos.TF.Denominator)  Y0=SkywalkerX8.InitialConditions.da  U0=SkywalkerX8.InitialConditions.da
  da : Outport
  wires:
  Rate Limiter/1 -> Saturation/1
  da*/1 -> Transfer Fcn (with initial outputs)/1
  Saturation/1 -> da/1
  Transfer Fcn (with initial outputs)/1 -> Rate Limiter/1

== system SkywalkerX8_Lateral_Control_Digital_Verification/Signal Builder ==
  Demux : Demux  Tag=STV Demux  Outputs=1
  FromWs : FromWorkspace  Tag=STV FromWs  VariableName=tuvar  SampleTime=0
      SigBuilderData=|
      | common.afterFinalStr = 'Extrapolate'
      | common.sampleTime = 0
      | dataSet.timeRange = [0 30]
      | dataSet.name = 'Group 1'
      | sbobj.Groups.Name = 'Group 1'
      | sbobj.Groups.Signals.Name = 'Signal 1'
      | sbobj.Groups.Signals.XData = [0 0.01 0.01 15 15 30]
      | sbobj.Groups.Signals.YData = [0 0 1.5708 1.5708 0 0]
      | sbobj.Groups.TimeRange = [0 30]
  Signal 1 : Outport  Tag=STV Outport
  wires:
  Demux/1 -> Signal 1/1
  FromWs/1 -> Demux/1

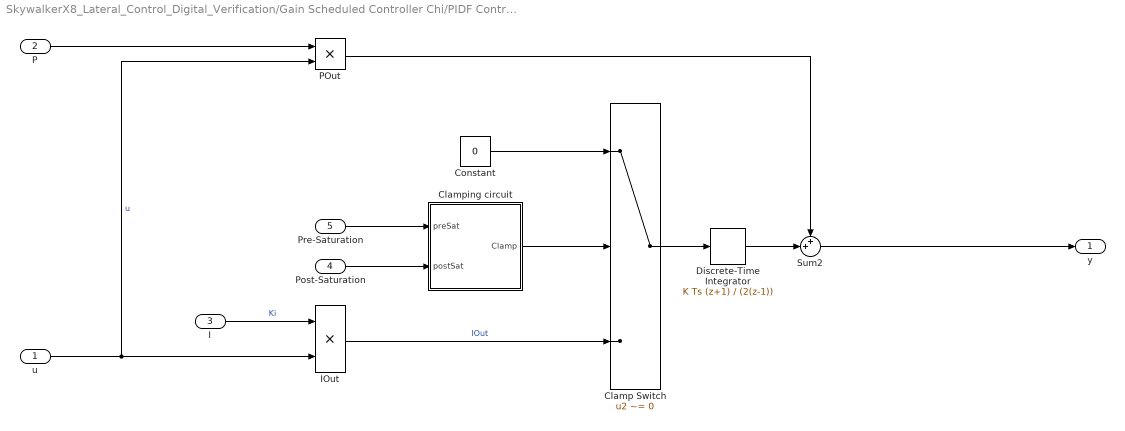
== system SkywalkerX8_Lateral_Control_Digital_Verification/Gain Scheduled Controller Chi/PIDF Controller Va_theta ==
  u : Inport
  P : Inport  Port=2
  I : Inport  Port=3
  Post-Saturation : Inport  Port=4
  Pre-Saturation : Inport  Port=5
  Clamp Switch : Switch  Criteria=u2 ~= 0
  Clamping circuit : Subsystem
  Constant : Constant  Value=0
  Discrete-Time Integrator : DiscreteIntegrator  IntegratorMethod=Integration: Trapezoidal  InitialCondition=SkywalkerX8.InitialConditions.PhiThetaPsi(1)  SampleTime=SkywalkerX8.Control.Lateral.ChiController.Digital.SampleTime  ICPrevOutput=DiscIntNeverNeededParam  ICPrevScaledInput=DiscIntNeverNeededParam
  IOut : Product  DisableCoverage=on
  POut : Product
  Sum2 : Sum  Inputs=++|
  y : Outport  InitialOutput=0
  wires:
  Sum2/1 -> y/1
  POut/1 -> Sum2/1
  u/1 -> POut/2, IOut/2  "u"
  Clamp Switch/1 -> Discrete-Time Integrator/1
  Discrete-Time Integrator/1 -> Sum2/2
  Constant/1 -> Clamp Switch/1
  I/1 -> IOut/1  "Ki"
  IOut/1 -> Clamp Switch/3  "IOut"
  Clamping circuit/1(Clamp) -> Clamp Switch/2
  P/1 -> POut/1
  Pre-Saturation/1 -> Clamping circuit/1(preSat)
  Post-Saturation/1 -> Clamping circuit/2(postSat)

== system SkywalkerX8_Lateral_Control_Digital_Verification/Gain Scheduled Controller Phi/DF Controller Phi ==
  N : Inport
  D : Inport  Port=2
  du/dt : Inport  Port=3
  Discrete-Time Integrator : DiscreteIntegrator  IntegratorMethod=Integration: Trapezoidal  SampleTime=SkywalkerX8.Control.Lateral.PhiController.Digital.SampleTime  ICPrevOutput=DiscIntNeverNeededParam  ICPrevScaledInput=DiscIntNeverNeededParam
  Product : Product
  Product1 : Product
  Sum : Sum  Inputs=|+-
  da* : Outport
  wires:
  Discrete-Time Integrator/1 -> da*/1, Sum/2  "da*"
  Product1/1 -> Discrete-Time Integrator/1  "Nda*_e"
  du/dt/1 -> Product/2
  D/1 -> Product/1
  Sum/1 -> Product1/2  "da*_e"
  N/1 -> Product1/1
  Product/1 -> Sum/1

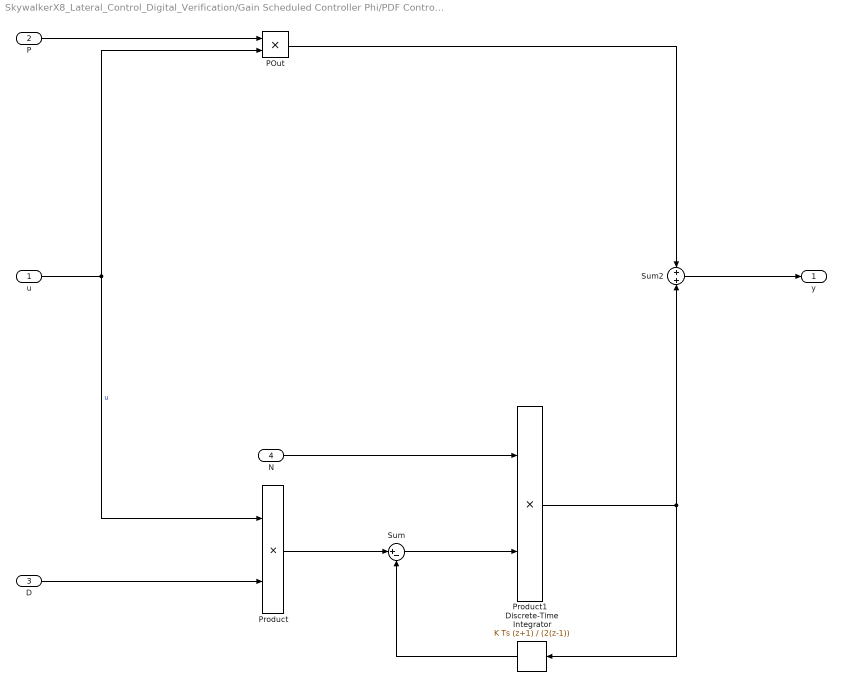
== system SkywalkerX8_Lateral_Control_Digital_Verification/Gain Scheduled Controller Phi/PDF Controller Phi 2DOF ==
  u : Inport
  P : Inport  Port=2
  D : Inport  Port=3
  N : Inport  Port=4
  Discrete-Time Integrator : DiscreteIntegrator  IntegratorMethod=Integration: Trapezoidal  SampleTime=SkywalkerX8.Control.Lateral.PhiController.Digital.SampleTime  ICPrevOutput=DiscIntNeverNeededParam  ICPrevScaledInput=DiscIntNeverNeededParam
  POut : Product
  Product : Product
  Product1 : Product
  Sum : Sum  Inputs=|+-
  Sum2 : Sum
  y : Outport  InitialOutput=0
  wires:
  Sum2/1 -> y/1
  N/1 -> Product1/1
  Product1/1 -> Discrete-Time Integrator/1, Sum2/2
  Sum/1 -> Product1/2
  POut/1 -> Sum2/1
  D/1 -> Product/2
  u/1 -> Product/1, POut/2  "u"
  Discrete-Time Integrator/1 -> Sum/2
  Product/1 -> Sum/1
  P/1 -> POut/1

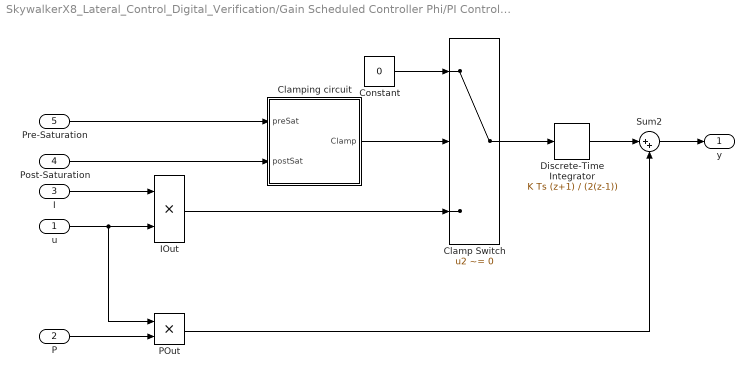
== system SkywalkerX8_Lateral_Control_Digital_Verification/Gain Scheduled Controller Phi/PI Controller Phi ==
  u : Inport
  P : Inport  Port=2
  I : Inport  Port=3
  Post-Saturation : Inport  Port=4
  Pre-Saturation : Inport  Port=5
  Clamp Switch : Switch  Criteria=u2 ~= 0
  Clamping circuit : Subsystem
  Constant : Constant  Value=0
  Discrete-Time Integrator : DiscreteIntegrator  IntegratorMethod=Integration: Trapezoidal  InitialCondition=SkywalkerX8.InitialConditions.da  SampleTime=SkywalkerX8.Control.Lateral.PhiController.Digital.SampleTime  ICPrevOutput=DiscIntNeverNeededParam  ICPrevScaledInput=DiscIntNeverNeededParam
  IOut : Product  DisableCoverage=on
  POut : Product
  Sum2 : Sum  Inputs=|++
  y : Outport  InitialOutput=0
  wires:
  IOut/1 -> Clamp Switch/3
  Clamp Switch/1 -> Discrete-Time Integrator/1
  Sum2/1 -> y/1
  Pre-Saturation/1 -> Clamping circuit/1(preSat)
  Post-Saturation/1 -> Clamping circuit/2(postSat)
  Clamping circuit/1(Clamp) -> Clamp Switch/2
  Constant/1 -> Clamp Switch/1
  Discrete-Time Integrator/1 -> Sum2/1
  POut/1 -> Sum2/2
  P/1 -> POut/2
  u/1 -> POut/1, IOut/2
  I/1 -> IOut/1

== system SkywalkerX8_Lateral_Control_Digital_Verification/Gain Scheduled Controller Theta/DF Controller Theta ==
  N : Inport
  D : Inport  Port=2
  du/dt : Inport  Port=3
  Discrete-Time Integrator : DiscreteIntegrator  IntegratorMethod=Integration: Trapezoidal  SampleTime=SkywalkerX8.Control.Longitudinal.thetaController.Digital.SampleTime  ICPrevOutput=DiscIntNeverNeededParam  ICPrevScaledInput=DiscIntNeverNeededParam
  Product : Product
  Product1 : Product
  Sum : Sum  Inputs=|+-
  de* : Outport
  wires:
  Discrete-Time Integrator/1 -> de*/1, Sum/2  "de*"
  Product1/1 -> Discrete-Time Integrator/1  "Nde*_e"
  du/dt/1 -> Product/2
  D/1 -> Product/1
  Sum/1 -> Product1/2  "de*_e"
  N/1 -> Product1/1
  Product/1 -> Sum/1

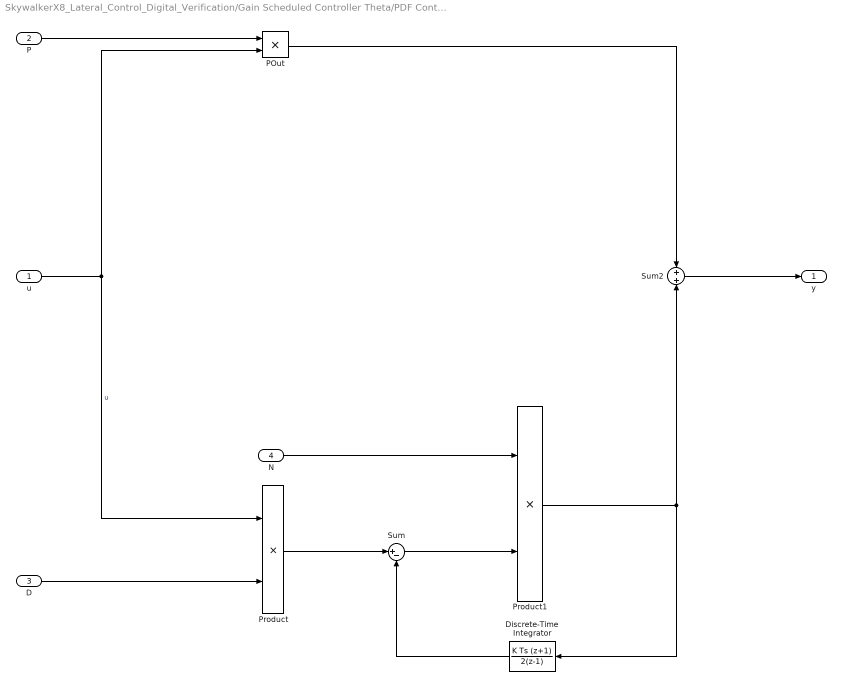
== system SkywalkerX8_Lateral_Control_Digital_Verification/Gain Scheduled Controller Theta/PDF Controller Theta 2DOF ==
  u : Inport
  P : Inport  Port=2
  D : Inport  Port=3
  N : Inport  Port=4
  Discrete-Time Integrator : DiscreteIntegrator  IntegratorMethod=Integration: Trapezoidal  SampleTime=SkywalkerX8.Control.Longitudinal.thetaController.Digital.SampleTime  ICPrevOutput=DiscIntNeverNeededParam  ICPrevScaledInput=DiscIntNeverNeededParam
  POut : Product
  Product : Product
  Product1 : Product
  Sum : Sum  Inputs=|+-
  Sum2 : Sum
  y : Outport  InitialOutput=0
  wires:
  Sum2/1 -> y/1
  N/1 -> Product1/1
  Product1/1 -> Discrete-Time Integrator/1, Sum2/2
  Sum/1 -> Product1/2
  POut/1 -> Sum2/1
  D/1 -> Product/2
  u/1 -> Product/1, POut/2  "u"
  Discrete-Time Integrator/1 -> Sum/2
  Product/1 -> Sum/1
  P/1 -> POut/1

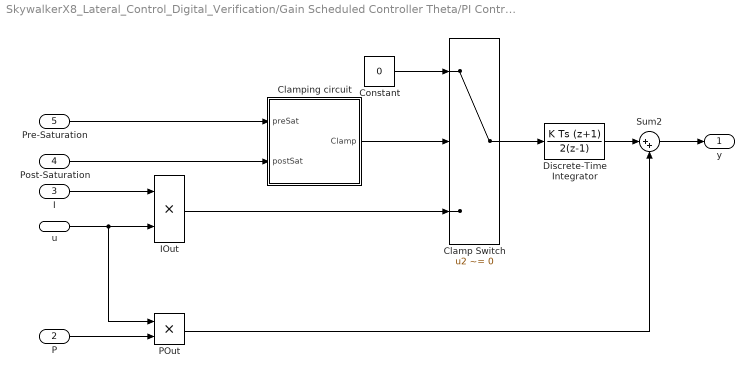
== system SkywalkerX8_Lateral_Control_Digital_Verification/Gain Scheduled Controller Theta/PI Controller Theta ==
  u : Inport
  P : Inport  Port=2
  I : Inport  Port=3
  Post-Saturation : Inport  Port=4
  Pre-Saturation : Inport  Port=5
  Clamp Switch : Switch  Criteria=u2 ~= 0
  Clamping circuit : Subsystem
  Constant : Constant  Value=0
  Discrete-Time Integrator : DiscreteIntegrator  IntegratorMethod=Integration: Trapezoidal  InitialCondition=SkywalkerX8.InitialConditions.ThetaController.Integrator  SampleTime=SkywalkerX8.Control.Longitudinal.thetaController.Digital.SampleTime  ICPrevOutput=DiscIntNeverNeededParam  ICPrevScaledInput=DiscIntNeverNeededParam
  IOut : Product  DisableCoverage=on
  POut : Product
  Sum2 : Sum  Inputs=|++
  y : Outport  InitialOutput=0
  wires:
  IOut/1 -> Clamp Switch/3
  Clamp Switch/1 -> Discrete-Time Integrator/1
  Sum2/1 -> y/1
  Pre-Saturation/1 -> Clamping circuit/1(preSat)
  Post-Saturation/1 -> Clamping circuit/2(postSat)
  Clamping circuit/1(Clamp) -> Clamp Switch/2
  Constant/1 -> Clamp Switch/1
  Discrete-Time Integrator/1 -> Sum2/1
  POut/1 -> Sum2/2
  P/1 -> POut/2
  u/1 -> POut/1, IOut/2
  I/1 -> IOut/1

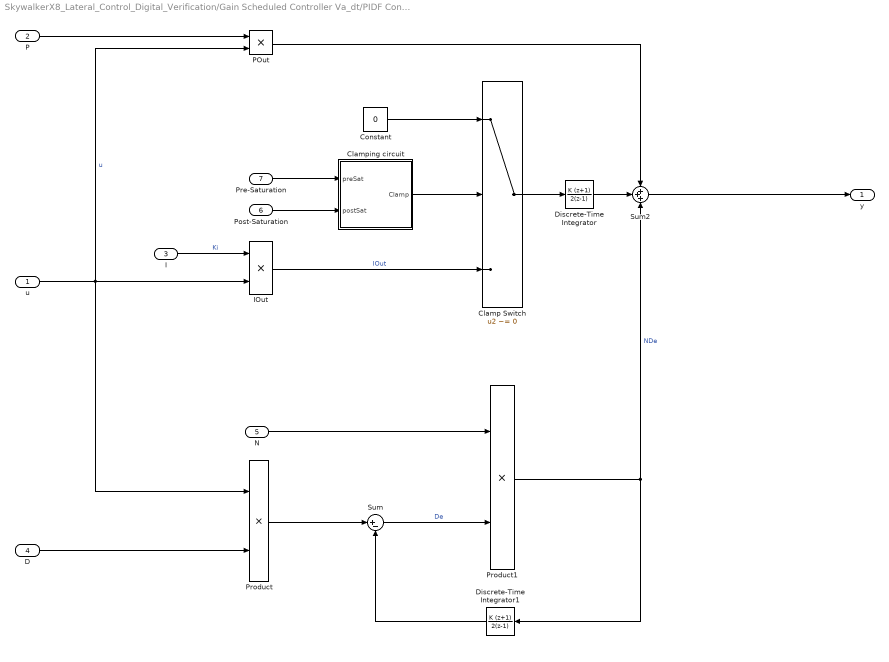
== system SkywalkerX8_Lateral_Control_Digital_Verification/Gain Scheduled Controller Va_dt/PIDF Controller Va_dt ==
  u : Inport
  P : Inport  Port=2
  I : Inport  Port=3
  D : Inport  Port=4
  N : Inport  Port=5
  Post-Saturation : Inport  Port=6
  Pre-Saturation : Inport  Port=7
  Clamp Switch : Switch  Criteria=u2 ~= 0
  Clamping circuit : Subsystem
  Constant : Constant  Value=0
  Discrete-Time Integrator : DiscreteIntegrator  IntegratorMethod=Accumulation: Trapezoidal  InitialCondition=SkywalkerX8.InitialConditions.dt  SampleTime=SkywalkerX8.Control.Longitudinal.VaDtController.Digital.SampleTime  ICPrevOutput=DiscIntNeverNeededParam  ICPrevScaledInput=DiscIntNeverNeededParam
  Discrete-Time Integrator1 : DiscreteIntegrator  IntegratorMethod=Accumulation: Trapezoidal  SampleTime=SkywalkerX8.Control.Longitudinal.VaDtController.Digital.SampleTime  ICPrevOutput=DiscIntNeverNeededParam  ICPrevScaledInput=DiscIntNeverNeededParam
  IOut : Product  DisableCoverage=on
  POut : Product
  Product : Product
  Product1 : Product
  Sum : Sum  Inputs=|+-
  Sum2 : Sum  Inputs=+++
  y : Outport  InitialOutput=0
  wires:
  Sum2/1 -> y/1
  N/1 -> Product1/1
  Product1/1 -> Discrete-Time Integrator1/1, Sum2/3  "NDe"
  Sum/1 -> Product1/2  "De"
  POut/1 -> Sum2/1
  D/1 -> Product/2
  u/1 -> POut/2, Product/1, IOut/2  "u"
  Discrete-Time Integrator1/1 -> Sum/2
  Clamp Switch/1 -> Discrete-Time Integrator/1
  Product/1 -> Sum/1
  Discrete-Time Integrator/1 -> Sum2/2
  Constant/1 -> Clamp Switch/1
  I/1 -> IOut/1  "Ki"
  IOut/1 -> Clamp Switch/3  "IOut"
  Clamping circuit/1(Clamp) -> Clamp Switch/2
  P/1 -> POut/1
  Pre-Saturation/1 -> Clamping circuit/1(preSat)
  Post-Saturation/1 -> Clamping circuit/2(postSat)

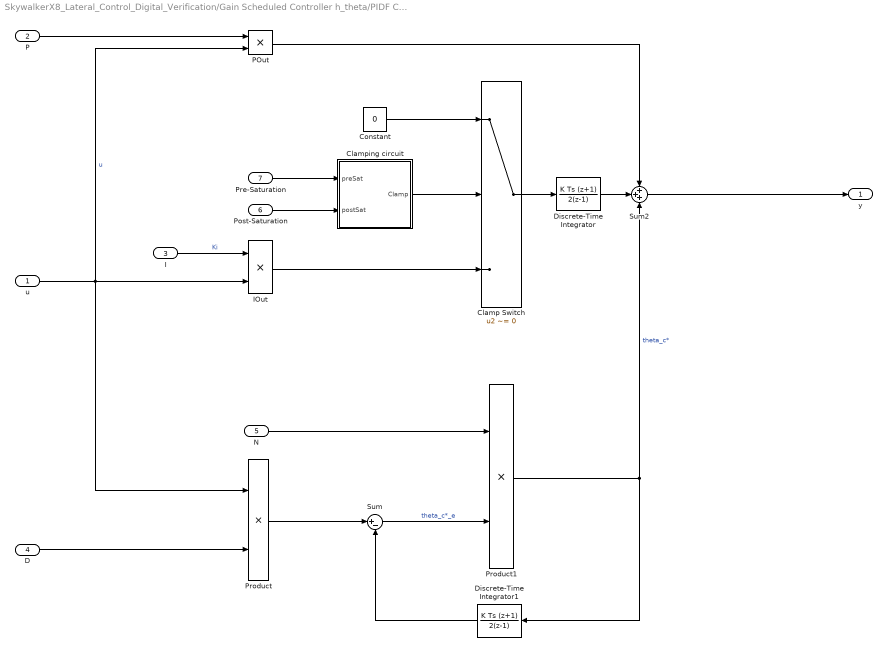
== system SkywalkerX8_Lateral_Control_Digital_Verification/Gain Scheduled Controller h_theta/PIDF Controller h_theta ==
  u : Inport
  P : Inport  Port=2
  I : Inport  Port=3
  D : Inport  Port=4
  N : Inport  Port=5
  Post-Saturation : Inport  Port=6
  Pre-Saturation : Inport  Port=7
  Clamp Switch : Switch  Criteria=u2 ~= 0
  Clamping circuit : Subsystem
  Constant : Constant  Value=0
  Discrete-Time Integrator : DiscreteIntegrator  IntegratorMethod=Integration: Trapezoidal  InitialCondition=SkywalkerX8.InitialConditions.PhiThetaPsi(2)  SampleTime=SkywalkerX8.Control.Longitudinal.altController.Digital.SampleTime  ICPrevOutput=DiscIntNeverNeededParam  ICPrevScaledInput=DiscIntNeverNeededParam
  Discrete-Time Integrator1 : DiscreteIntegrator  IntegratorMethod=Integration: Trapezoidal  SampleTime=SkywalkerX8.Control.Longitudinal.altController.Digital.SampleTime  ICPrevOutput=DiscIntNeverNeededParam  ICPrevScaledInput=DiscIntNeverNeededParam
  IOut : Product  DisableCoverage=on
  POut : Product
  Product : Product
  Product1 : Product
  Sum : Sum  Inputs=|+-
  Sum2 : Sum  Inputs=+++
  y : Outport  InitialOutput=0
  wires:
  Sum2/1 -> y/1
  N/1 -> Product1/1
  Product1/1 -> Discrete-Time Integrator1/1, Sum2/3  "theta_c*"
  Sum/1 -> Product1/2  "theta_c*_e"
  POut/1 -> Sum2/1
  D/1 -> Product/2
  u/1 -> POut/2, Product/1, IOut/2  "u"
  Discrete-Time Integrator1/1 -> Sum/2
  Clamp Switch/1 -> Discrete-Time Integrator/1
  Product/1 -> Sum/1
  Discrete-Time Integrator/1 -> Sum2/2
  Constant/1 -> Clamp Switch/1
  I/1 -> IOut/1  "Ki"
  IOut/1 -> Clamp Switch/3
  Clamping circuit/1(Clamp) -> Clamp Switch/2
  P/1 -> POut/1
  Pre-Saturation/1 -> Clamping circuit/1(preSat)
  Post-Saturation/1 -> Clamping circuit/2(postSat)

== system SkywalkerX8_Lateral_Control_Digital_Verification/Gain Scheduled Controller Chi/PIDF Controller Va_theta/Clamping circuit ==
  preSat : Inport  DisableCoverage=on
  postSat : Inport  DisableCoverage=on  Port=2
  Memory : Memory  DisableCoverage=on
  NotEqual : RelationalOperator  DisableCoverage=on  Operator=~=  RndMeth=Nearest  InputSameDT=on
  Clamp : Outport  DisableCoverage=on
  wires:
  postSat/1 -> NotEqual/2
  preSat/1 -> NotEqual/1
  NotEqual/1 -> Memory/1
  Memory/1 -> Clamp/1

== system SkywalkerX8_Lateral_Control_Digital_Verification/Gain Scheduled Controller Phi/PI Controller Phi/Clamping circuit ==
  preSat : Inport  DisableCoverage=on
  postSat : Inport  DisableCoverage=on  Port=2
  Memory : Memory  DisableCoverage=on
  NotEqual : RelationalOperator  DisableCoverage=on  Operator=~=  RndMeth=Nearest  InputSameDT=on
  Clamp : Outport  DisableCoverage=on
  wires:
  postSat/1 -> NotEqual/2
  preSat/1 -> NotEqual/1
  NotEqual/1 -> Memory/1
  Memory/1 -> Clamp/1

== system SkywalkerX8_Lateral_Control_Digital_Verification/Gain Scheduled Controller Theta/PI Controller Theta/Clamping circuit ==
  preSat : Inport  DisableCoverage=on
  postSat : Inport  DisableCoverage=on  Port=2
  Memory : Memory  DisableCoverage=on
  NotEqual : RelationalOperator  DisableCoverage=on  Operator=~=  RndMeth=Nearest  InputSameDT=on
  Clamp : Outport  DisableCoverage=on
  wires:
  postSat/1 -> NotEqual/2
  preSat/1 -> NotEqual/1
  NotEqual/1 -> Memory/1
  Memory/1 -> Clamp/1

== system SkywalkerX8_Lateral_Control_Digital_Verification/Gain Scheduled Controller Va_dt/PIDF Controller Va_dt/Clamping circuit ==
  preSat : Inport  DisableCoverage=on
  postSat : Inport  DisableCoverage=on  Port=2
  Memory : Memory  DisableCoverage=on
  NotEqual : RelationalOperator  DisableCoverage=on  Operator=~=  RndMeth=Nearest  InputSameDT=on
  Clamp : Outport  DisableCoverage=on
  wires:
  postSat/1 -> NotEqual/2
  preSat/1 -> NotEqual/1
  NotEqual/1 -> Memory/1
  Memory/1 -> Clamp/1

== system SkywalkerX8_Lateral_Control_Digital_Verification/Gain Scheduled Controller h_theta/PIDF Controller h_theta/Clamping circuit ==
  preSat : Inport  DisableCoverage=on
  postSat : Inport  DisableCoverage=on  Port=2
  Memory : Memory  DisableCoverage=on
  NotEqual : RelationalOperator  DisableCoverage=on  Operator=~=  RndMeth=Nearest  InputSameDT=on
  Clamp : Outport  DisableCoverage=on
  wires:
  postSat/1 -> NotEqual/2
  preSat/1 -> NotEqual/1
  NotEqual/1 -> Memory/1
  Memory/1 -> Clamp/1
